simulink model "MiniDAQ"  (R2022a)
settings: Solver=FixedStepAuto  StartTime=0.0  StopTime=3660  FixedStep=Ts  RelTol=1e-3
undefined symbols (not defined in the file or in its folder): ADC, ADC1, ADC2, ADC3, ADC4, ax, ay, az, IMU, pitch, roll, yaw
libraries: slrealtimeethercatlib x33, slrealtimeloglib x1
settings Model: SimulationMode=external  Creator=Bret  LastModifiedBy=HWRL user
settings SolverCC: ConcurrentTasks=on  AlgebraicLoopSolver=TrustRegion  PositivePriorityOrder=on
settings OptimizationCC: BlockReduction=off  OptimizeBlockIOStorage=off
settings DebuggingCC: TasksWithSamePriorityMsg=none  ParameterPrecisionLossMsg=none  UnconnectedInputMsg=warning  UnconnectedOutputMsg=warning  UnconnectedLineMsg=warning  SFMachineParentedDataDiag=warning
settings HardwareCC: ProdBitPerLong=64  ProdLongLongMode=on  ProdHWDeviceType=Intel->x86-64 (Linux 64)
settings RTWCC: Description=Simulink Real-Time  SystemTargetFile=slrealtime.tlc  TemplateMakefile=slrealtime_default_tmf  RTWVerbose=off  Toolchain=Simulink Real-Time Toolchain  BuildConfiguration=Faster Runs  CodeExecutionProfiling=on  TargetLang=C++  DLArmComputeVersion=19.05
settings SimulinkRealTimeTargetCC: UseGCCFastMath=on

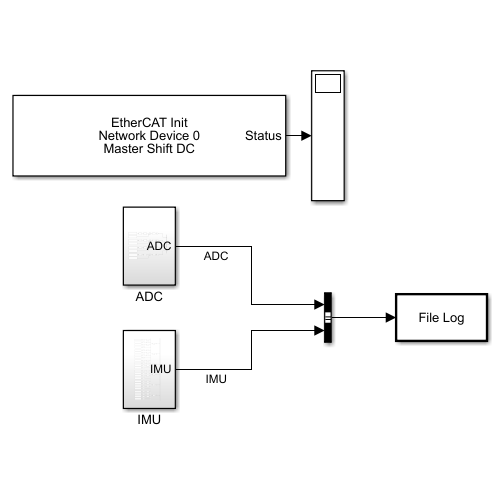
[thumbnail: Simulink's stored preview of the top-level diagram]
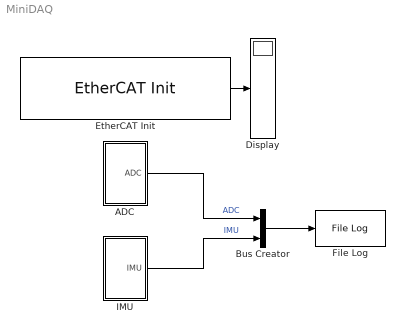
== system MiniDAQ ==
  ADC : Subsystem
  Bus Creator : BusCreator  Inputs=ADC,IMU
  Display : Display
  EtherCAT Init : slrealtimeethercatlib/EtherCAT Init  Priority=0  config_file=C:\Software\Mini-DAQ\TwinCAT\MiniDAQ1kHzDC.xml  device_id=0  pci_bus=0  pci_slot=0  pci_function=0  portnum=1  initstate=2  dctuning=0  enaDebug=0  enaDC=on  errLink=off  masterDbg=off  stateChgDbg=off  baseClock=off  masterCfg=off  logFile='c:\dbglog.txt'  sample_time=0.001000  DCMode=2
      settings: SourceProductBaseCode=XP
  File Log : slrealtimeloglib/File Log  decimation=1  inputProcessing=Elements as channels (sample based)
      settings: SourceProductBaseCode=XP
  IMU : Subsystem
  wires:
  EtherCAT Init/1 -> Display/1
  Bus Creator/1 -> File Log/1
  ADC/1(ADC) -> Bus Creator/1  "ADC"
  IMU/1(IMU) -> Bus Creator/2  "IMU"

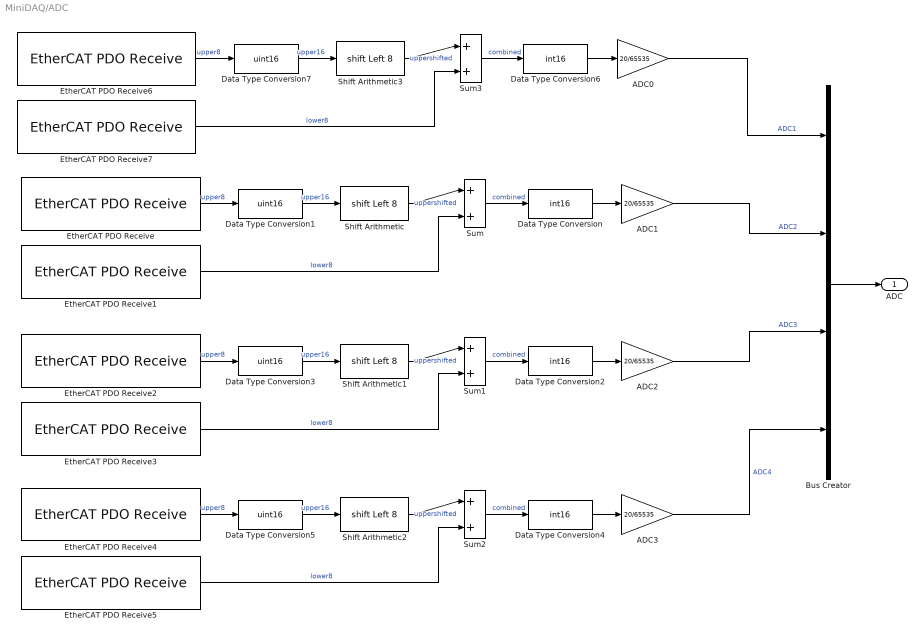
== system MiniDAQ/ADC ==
  ADC{0..3} (4 alike) : Gain  Gain=20/65535  OutDataTypeStr=double
  Bus Creator : BusCreator  Inputs=ADC1,ADC2,ADC3,ADC4
  Data Type Conversion{,2,4,6} (4 alike) : DataTypeConversion  OutDataTypeStr=int16  SaturateOnIntegerOverflow=off  RndMeth=Floor
  Data Type Conversion{1,3,5,7} (4 alike) : DataTypeConversion  OutDataTypeStr=uint16  SaturateOnIntegerOverflow=off  RndMeth=Floor
  EtherCAT PDO Receive : slrealtimeethercatlib/EtherCAT PDO Receive  Priority=2  sig_name=Box 1 (EasyCAT 32+32 rev 1).Inputs.Byte2  sig_offset=480  sig_type=uint8  type_size=8  sig_dim=1  device_id=0  sample_time=0.001000
      settings: SourceProductBaseCode=XP
  EtherCAT PDO Receive1 : slrealtimeethercatlib/EtherCAT PDO Receive  Priority=2  sig_name=Box 1 (EasyCAT 32+32 rev 1).Inputs.Byte3  sig_offset=488  sig_type=uint8  type_size=8  sig_dim=1  device_id=0  sample_time=0.001000
      settings: SourceProductBaseCode=XP
  EtherCAT PDO Receive2 : slrealtimeethercatlib/EtherCAT PDO Receive  Priority=2  sig_name=Box 1 (EasyCAT 32+32 rev 1).Inputs.Byte4  sig_offset=496  sig_type=uint8  type_size=8  sig_dim=1  device_id=0  sample_time=0.001000
      settings: SourceProductBaseCode=XP
  EtherCAT PDO Receive3 : slrealtimeethercatlib/EtherCAT PDO Receive  Priority=2  sig_name=Box 1 (EasyCAT 32+32 rev 1).Inputs.Byte5  sig_offset=504  sig_type=uint8  type_size=8  sig_dim=1  device_id=0  sample_time=0.001000
      settings: SourceProductBaseCode=XP
  EtherCAT PDO Receive4 : slrealtimeethercatlib/EtherCAT PDO Receive  Priority=2  sig_name=Box 1 (EasyCAT 32+32 rev 1).Inputs.Byte6  sig_offset=512  sig_type=uint8  type_size=8  sig_dim=1  device_id=0  sample_time=0.001000
      settings: SourceProductBaseCode=XP
  EtherCAT PDO Receive5 : slrealtimeethercatlib/EtherCAT PDO Receive  Priority=2  sig_name=Box 1 (EasyCAT 32+32 rev 1).Inputs.Byte7  sig_offset=520  sig_type=uint8  type_size=8  sig_dim=1  device_id=0  sample_time=0.001000
      settings: SourceProductBaseCode=XP
  EtherCAT PDO Receive6 : slrealtimeethercatlib/EtherCAT PDO Receive  Priority=2  sig_name=Box 1 (EasyCAT 32+32 rev 1).Inputs.Byte0  sig_offset=464  sig_type=uint8  type_size=8  sig_dim=1  device_id=0  sample_time=0.001000
      settings: SourceProductBaseCode=XP
  EtherCAT PDO Receive7 : slrealtimeethercatlib/EtherCAT PDO Receive  Priority=2  sig_name=Box 1 (EasyCAT 32+32 rev 1).Inputs.Byte1  sig_offset=472  sig_type=uint8  type_size=8  sig_dim=1  device_id=0  sample_time=0.001000
      settings: SourceProductBaseCode=XP
  Shift Arithmetic{,1..3} (4 alike) : ArithShift  BitShiftNumber=8  BitShiftDirection=Left
  Sum{,1..3} (4 alike) : Sum  Inputs=|++
  ADC : Outport
  wires:
  ADC1/1 -> Bus Creator/2  "ADC2"
  Sum/1 -> Data Type Conversion/1  "combined"
  Data Type Conversion1/1 -> Shift Arithmetic/1  "upper16"
  Shift Arithmetic/1 -> Sum/1  "uppershifted"
  Data Type Conversion/1 -> ADC1/1
  EtherCAT PDO Receive/1 -> Data Type Conversion1/1  "upper8"
  EtherCAT PDO Receive1/1 -> Sum/2  "lower8"
  EtherCAT PDO Receive3/1 -> Sum1/2  "lower8"
  EtherCAT PDO Receive2/1 -> Data Type Conversion3/1  "upper8"
  Data Type Conversion2/1 -> ADC2/1
  Shift Arithmetic1/1 -> Sum1/1  "uppershifted"
  Data Type Conversion3/1 -> Shift Arithmetic1/1  "upper16"
  Sum1/1 -> Data Type Conversion2/1  "combined"
  ADC2/1 -> Bus Creator/3  "ADC3"
  ADC3/1 -> Bus Creator/4  "ADC4"
  Sum2/1 -> Data Type Conversion4/1  "combined"
  Data Type Conversion5/1 -> Shift Arithmetic2/1  "upper16"
  Shift Arithmetic2/1 -> Sum2/1  "uppershifted"
  Data Type Conversion4/1 -> ADC3/1
  EtherCAT PDO Receive4/1 -> Data Type Conversion5/1  "upper8"
  EtherCAT PDO Receive5/1 -> Sum2/2  "lower8"
  EtherCAT PDO Receive7/1 -> Sum3/2  "lower8"
  EtherCAT PDO Receive6/1 -> Data Type Conversion7/1  "upper8"
  Data Type Conversion6/1 -> ADC0/1
  Shift Arithmetic3/1 -> Sum3/1  "uppershifted"
  Data Type Conversion7/1 -> Shift Arithmetic3/1  "upper16"
  Sum3/1 -> Data Type Conversion6/1  "combined"
  ADC0/1 -> Bus Creator/1  "ADC1"
  Bus Creator/1 -> ADC/1

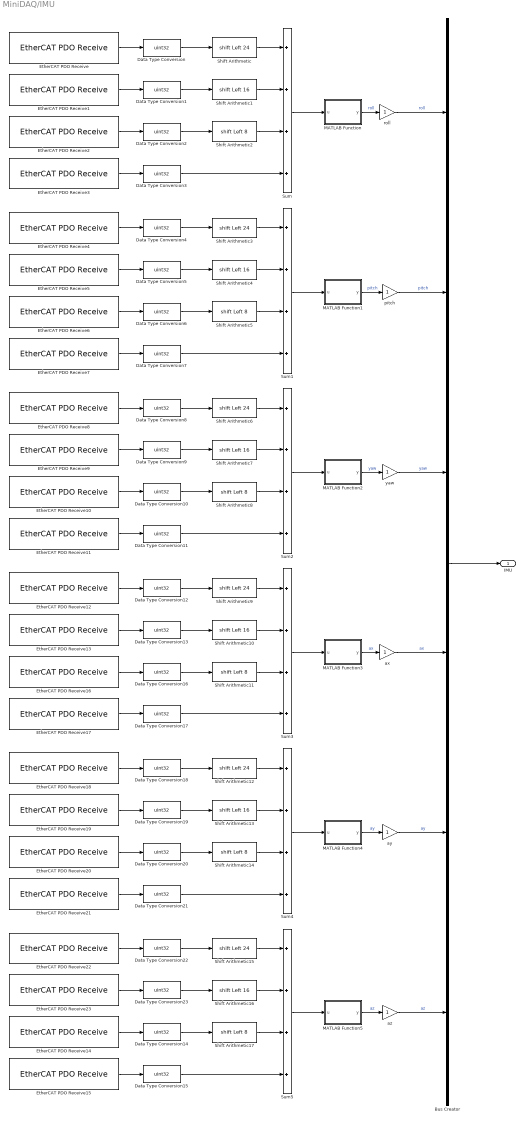
== system MiniDAQ/IMU ==
  Bus Creator : BusCreator  Inputs=roll,pitch,yaw,ax,ay,az
  Data Type Conversion{,1..23} (24 alike) : DataTypeConversion  OutDataTypeStr=uint32  SaturateOnIntegerOverflow=off  RndMeth=Floor
  EtherCAT PDO Receive : slrealtimeethercatlib/EtherCAT PDO Receive  Priority=2  sig_name=Box 1 (EasyCAT 32+32 rev 1).Inputs.Byte8  sig_offset=528  sig_type=uint8  type_size=8  sig_dim=1  device_id=0  sample_time=0.001000
      settings: SourceProductBaseCode=XP
  EtherCAT PDO Receive1 : slrealtimeethercatlib/EtherCAT PDO Receive  Priority=2  sig_name=Box 1 (EasyCAT 32+32 rev 1).Inputs.Byte9  sig_offset=536  sig_type=uint8  type_size=8  sig_dim=1  device_id=0  sample_time=0.001000
      settings: SourceProductBaseCode=XP
  EtherCAT PDO Receive10 : slrealtimeethercatlib/EtherCAT PDO Receive  Priority=2  sig_name=Box 1 (EasyCAT 32+32 rev 1).Inputs.Byte18  sig_offset=608  sig_type=uint8  type_size=8  sig_dim=1  device_id=0  sample_time=0.001000
      settings: SourceProductBaseCode=XP
  EtherCAT PDO Receive11 : slrealtimeethercatlib/EtherCAT PDO Receive  Priority=2  sig_name=Box 1 (EasyCAT 32+32 rev 1).Inputs.Byte19  sig_offset=616  sig_type=uint8  type_size=8  sig_dim=1  device_id=0  sample_time=0.001000
      settings: SourceProductBaseCode=XP
  EtherCAT PDO Receive12 : slrealtimeethercatlib/EtherCAT PDO Receive  Priority=2  sig_name=Box 1 (EasyCAT 32+32 rev 1).Inputs.Byte20  sig_offset=624  sig_type=uint8  type_size=8  sig_dim=1  device_id=0  sample_time=0.001000
      settings: SourceProductBaseCode=XP
  EtherCAT PDO Receive13 : slrealtimeethercatlib/EtherCAT PDO Receive  Priority=2  sig_name=Box 1 (EasyCAT 32+32 rev 1).Inputs.Byte21  sig_offset=632  sig_type=uint8  type_size=8  sig_dim=1  device_id=0  sample_time=0.001000
      settings: SourceProductBaseCode=XP
  EtherCAT PDO Receive14 : slrealtimeethercatlib/EtherCAT PDO Receive  Priority=2  sig_name=Box 1 (EasyCAT 32+32 rev 1).Inputs.Byte30  sig_offset=704  sig_type=uint8  type_size=8  sig_dim=1  device_id=0  sample_time=0.001000
      settings: SourceProductBaseCode=XP
  EtherCAT PDO Receive15 : slrealtimeethercatlib/EtherCAT PDO Receive  Priority=2  sig_name=Box 1 (EasyCAT 32+32 rev 1).Inputs.Byte31  sig_offset=712  sig_type=uint8  type_size=8  sig_dim=1  device_id=0  sample_time=0.001000
      settings: SourceProductBaseCode=XP
  EtherCAT PDO Receive16 : slrealtimeethercatlib/EtherCAT PDO Receive  Priority=2  sig_name=Box 1 (EasyCAT 32+32 rev 1).Inputs.Byte22  sig_offset=640  sig_type=uint8  type_size=8  sig_dim=1  device_id=0  sample_time=0.001000
      settings: SourceProductBaseCode=XP
  EtherCAT PDO Receive17 : slrealtimeethercatlib/EtherCAT PDO Receive  Priority=2  sig_name=Box 1 (EasyCAT 32+32 rev 1).Inputs.Byte23  sig_offset=648  sig_type=uint8  type_size=8  sig_dim=1  device_id=0  sample_time=0.001000
      settings: SourceProductBaseCode=XP
  EtherCAT PDO Receive18 : slrealtimeethercatlib/EtherCAT PDO Receive  Priority=2  sig_name=Box 1 (EasyCAT 32+32 rev 1).Inputs.Byte24  sig_offset=656  sig_type=uint8  type_size=8  sig_dim=1  device_id=0  sample_time=0.001000
      settings: SourceProductBaseCode=XP
  EtherCAT PDO Receive19 : slrealtimeethercatlib/EtherCAT PDO Receive  Priority=2  sig_name=Box 1 (EasyCAT 32+32 rev 1).Inputs.Byte25  sig_offset=664  sig_type=uint8  type_size=8  sig_dim=1  device_id=0  sample_time=0.001000
      settings: SourceProductBaseCode=XP
  EtherCAT PDO Receive2 : slrealtimeethercatlib/EtherCAT PDO Receive  Priority=2  sig_name=Box 1 (EasyCAT 32+32 rev 1).Inputs.Byte10  sig_offset=544  sig_type=uint8  type_size=8  sig_dim=1  device_id=0  sample_time=0.001000
      settings: SourceProductBaseCode=XP
  EtherCAT PDO Receive20 : slrealtimeethercatlib/EtherCAT PDO Receive  Priority=2  sig_name=Box 1 (EasyCAT 32+32 rev 1).Inputs.Byte26  sig_offset=672  sig_type=uint8  type_size=8  sig_dim=1  device_id=0  sample_time=0.001000
      settings: SourceProductBaseCode=XP
  EtherCAT PDO Receive21 : slrealtimeethercatlib/EtherCAT PDO Receive  Priority=2  sig_name=Box 1 (EasyCAT 32+32 rev 1).Inputs.Byte27  sig_offset=680  sig_type=uint8  type_size=8  sig_dim=1  device_id=0  sample_time=0.001000
      settings: SourceProductBaseCode=XP
  EtherCAT PDO Receive22 : slrealtimeethercatlib/EtherCAT PDO Receive  Priority=2  sig_name=Box 1 (EasyCAT 32+32 rev 1).Inputs.Byte28  sig_offset=688  sig_type=uint8  type_size=8  sig_dim=1  device_id=0  sample_time=0.001000
      settings: SourceProductBaseCode=XP
  EtherCAT PDO Receive23 : slrealtimeethercatlib/EtherCAT PDO Receive  Priority=2  sig_name=Box 1 (EasyCAT 32+32 rev 1).Inputs.Byte29  sig_offset=696  sig_type=uint8  type_size=8  sig_dim=1  device_id=0  sample_time=0.001000
      settings: SourceProductBaseCode=XP
  EtherCAT PDO Receive3 : slrealtimeethercatlib/EtherCAT PDO Receive  Priority=2  sig_name=Box 1 (EasyCAT 32+32 rev 1).Inputs.Byte11  sig_offset=552  sig_type=uint8  type_size=8  sig_dim=1  device_id=0  sample_time=0.001000
      settings: SourceProductBaseCode=XP
  EtherCAT PDO Receive4 : slrealtimeethercatlib/EtherCAT PDO Receive  Priority=2  sig_name=Box 1 (EasyCAT 32+32 rev 1).Inputs.Byte12  sig_offset=560  sig_type=uint8  type_size=8  sig_dim=1  device_id=0  sample_time=0.001000
      settings: SourceProductBaseCode=XP
  EtherCAT PDO Receive5 : slrealtimeethercatlib/EtherCAT PDO Receive  Priority=2  sig_name=Box 1 (EasyCAT 32+32 rev 1).Inputs.Byte13  sig_offset=568  sig_type=uint8  type_size=8  sig_dim=1  device_id=0  sample_time=0.001000
      settings: SourceProductBaseCode=XP
  EtherCAT PDO Receive6 : slrealtimeethercatlib/EtherCAT PDO Receive  Priority=2  sig_name=Box 1 (EasyCAT 32+32 rev 1).Inputs.Byte14  sig_offset=576  sig_type=uint8  type_size=8  sig_dim=1  device_id=0  sample_time=0.001000
      settings: SourceProductBaseCode=XP
  EtherCAT PDO Receive7 : slrealtimeethercatlib/EtherCAT PDO Receive  Priority=2  sig_name=Box 1 (EasyCAT 32+32 rev 1).Inputs.Byte15  sig_offset=584  sig_type=uint8  type_size=8  sig_dim=1  device_id=0  sample_time=0.001000
      settings: SourceProductBaseCode=XP
  EtherCAT PDO Receive8 : slrealtimeethercatlib/EtherCAT PDO Receive  Priority=2  sig_name=Box 1 (EasyCAT 32+32 rev 1).Inputs.Byte16  sig_offset=592  sig_type=uint8  type_size=8  sig_dim=1  device_id=0  sample_time=0.001000
      settings: SourceProductBaseCode=XP
  EtherCAT PDO Receive9 : slrealtimeethercatlib/EtherCAT PDO Receive  Priority=2  sig_name=Box 1 (EasyCAT 32+32 rev 1).Inputs.Byte17  sig_offset=600  sig_type=uint8  type_size=8  sig_dim=1  device_id=0  sample_time=0.001000
      settings: SourceProductBaseCode=XP
  MATLAB Function : MATLAB Function  TreatAsAtomicUnit=on
  MATLAB Function1 : MATLAB Function  TreatAsAtomicUnit=on
  MATLAB Function2 : MATLAB Function  TreatAsAtomicUnit=on
  MATLAB Function3 : MATLAB Function  TreatAsAtomicUnit=on
  MATLAB Function4 : MATLAB Function  TreatAsAtomicUnit=on
  MATLAB Function5 : MATLAB Function  TreatAsAtomicUnit=on
  Shift Arithmetic{,3,6,9,12,15} (6 alike) : ArithShift  BitShiftNumber=24  BitShiftDirection=Left
  Shift Arithmetic{1,4,7,10,13,16} (6 alike) : ArithShift  BitShiftNumber=16  BitShiftDirection=Left
  Shift Arithmetic{2,5,8,11,14,17} (6 alike) : ArithShift  BitShiftNumber=8  BitShiftDirection=Left
  Sum{,1..5} (6 alike) : Sum  Inputs=++++
  ax : Gain  OutDataTypeStr=double
  ay : Gain  OutDataTypeStr=double
  az : Gain  OutDataTypeStr=double
  pitch : Gain  OutDataTypeStr=double
  roll : Gain  OutDataTypeStr=double
  yaw : Gain  OutDataTypeStr=double
  IMU : Outport
  wires:
  EtherCAT PDO Receive/1 -> Data Type Conversion/1
  EtherCAT PDO Receive1/1 -> Data Type Conversion1/1
  EtherCAT PDO Receive2/1 -> Data Type Conversion2/1
  EtherCAT PDO Receive3/1 -> Data Type Conversion3/1
  Data Type Conversion/1 -> Shift Arithmetic/1
  Data Type Conversion1/1 -> Shift Arithmetic1/1
  Data Type Conversion2/1 -> Shift Arithmetic2/1
  Shift Arithmetic/1 -> Sum/1
  Shift Arithmetic1/1 -> Sum/2
  Shift Arithmetic2/1 -> Sum/3
  Data Type Conversion3/1 -> Sum/4
  Sum/1 -> MATLAB Function/1(u)
  Bus Creator/1 -> IMU/1
  roll/1 -> Bus Creator/1  "roll"
  MATLAB Function1/1(y) -> pitch/1  "pitch"
  Sum1/1 -> MATLAB Function1/1(u)
  Data Type Conversion7/1 -> Sum1/4
  Shift Arithmetic5/1 -> Sum1/3
  Shift Arithmetic4/1 -> Sum1/2
  Shift Arithmetic3/1 -> Sum1/1
  Data Type Conversion6/1 -> Shift Arithmetic5/1
  Data Type Conversion5/1 -> Shift Arithmetic4/1
  Data Type Conversion4/1 -> Shift Arithmetic3/1
  EtherCAT PDO Receive7/1 -> Data Type Conversion7/1
  EtherCAT PDO Receive6/1 -> Data Type Conversion6/1
  EtherCAT PDO Receive5/1 -> Data Type Conversion5/1
  EtherCAT PDO Receive4/1 -> Data Type Conversion4/1
  MATLAB Function/1(y) -> roll/1  "roll"
  pitch/1 -> Bus Creator/2  "pitch"
  yaw/1 -> Bus Creator/3  "yaw"
  EtherCAT PDO Receive8/1 -> Data Type Conversion8/1
  EtherCAT PDO Receive9/1 -> Data Type Conversion9/1
  EtherCAT PDO Receive10/1 -> Data Type Conversion10/1
  EtherCAT PDO Receive11/1 -> Data Type Conversion11/1
  Data Type Conversion8/1 -> Shift Arithmetic6/1
  Data Type Conversion9/1 -> Shift Arithmetic7/1
  Data Type Conversion10/1 -> Shift Arithmetic8/1
  Shift Arithmetic6/1 -> Sum2/1
  Shift Arithmetic7/1 -> Sum2/2
  Shift Arithmetic8/1 -> Sum2/3
  Data Type Conversion11/1 -> Sum2/4
  Sum2/1 -> MATLAB Function2/1(u)
  MATLAB Function2/1(y) -> yaw/1  "yaw"
  MATLAB Function5/1(y) -> az/1  "az"
  Sum5/1 -> MATLAB Function5/1(u)
  Data Type Conversion15/1 -> Sum5/4
  Shift Arithmetic17/1 -> Sum5/3
  Shift Arithmetic16/1 -> Sum5/2
  Shift Arithmetic15/1 -> Sum5/1
  Data Type Conversion14/1 -> Shift Arithmetic17/1
  Data Type Conversion23/1 -> Shift Arithmetic16/1
  Data Type Conversion22/1 -> Shift Arithmetic15/1
  EtherCAT PDO Receive15/1 -> Data Type Conversion15/1
  EtherCAT PDO Receive14/1 -> Data Type Conversion14/1
  EtherCAT PDO Receive23/1 -> Data Type Conversion23/1
  EtherCAT PDO Receive22/1 -> Data Type Conversion22/1
  MATLAB Function3/1(y) -> ax/1  "ax"
  EtherCAT PDO Receive18/1 -> Data Type Conversion18/1
  EtherCAT PDO Receive19/1 -> Data Type Conversion19/1
  EtherCAT PDO Receive20/1 -> Data Type Conversion20/1
  EtherCAT PDO Receive21/1 -> Data Type Conversion21/1
  Data Type Conversion18/1 -> Shift Arithmetic12/1
  Data Type Conversion19/1 -> Shift Arithmetic13/1
  Data Type Conversion20/1 -> Shift Arithmetic14/1
  Shift Arithmetic12/1 -> Sum4/1
  Shift Arithmetic13/1 -> Sum4/2
  Shift Arithmetic14/1 -> Sum4/3
  Data Type Conversion21/1 -> Sum4/4
  Sum4/1 -> MATLAB Function4/1(u)
  MATLAB Function4/1(y) -> ay/1  "ay"
  ax/1 -> Bus Creator/4  "ax"
  Sum3/1 -> MATLAB Function3/1(u)
  Data Type Conversion17/1 -> Sum3/4
  Shift Arithmetic11/1 -> Sum3/3
  Shift Arithmetic10/1 -> Sum3/2
  Shift Arithmetic9/1 -> Sum3/1
  Data Type Conversion16/1 -> Shift Arithmetic11/1
  Data Type Conversion13/1 -> Shift Arithmetic10/1
  Data Type Conversion12/1 -> Shift Arithmetic9/1
  EtherCAT PDO Receive17/1 -> Data Type Conversion17/1
  EtherCAT PDO Receive16/1 -> Data Type Conversion16/1
  EtherCAT PDO Receive13/1 -> Data Type Conversion13/1
  EtherCAT PDO Receive12/1 -> Data Type Conversion12/1
  ay/1 -> Bus Creator/5  "ay"
  az/1 -> Bus Creator/6  "az"

== matlab function MiniDAQ/IMU/MATLAB Function ==
  data: u input; y output
function y = fcn(u)
y = typecast(u,'single');

== matlab function MiniDAQ/IMU/MATLAB Function2 ==
  data: u input; y output
function y = fcn(u)
y = typecast(u,'single');

== matlab function MiniDAQ/IMU/MATLAB Function3 ==
  data: u input; y output
function y = fcn(u)
y = typecast(u,'single');

== matlab function MiniDAQ/IMU/MATLAB Function4 ==
  data: u input; y output
function y = fcn(u)
y = typecast(u,'single');

== matlab function MiniDAQ/IMU/MATLAB Function5 ==
  data: u input; y output
function y = fcn(u)
y = typecast(u,'single');

== matlab function MiniDAQ/IMU/MATLAB Function1 ==
  data: u input; y output
function y = fcn(u)
y = typecast(u,'single');
